simulink subsystem "brakeRegen"  (R2022b)
settings: Solver=VariableStepAuto  StartTime=0.0  StopTime=10.0  RelTol=1e-3
libraries: brakeRegen_lib x1, Raptor_lib x1
settings Model: Creator=serga  LastModifiedBy=serga

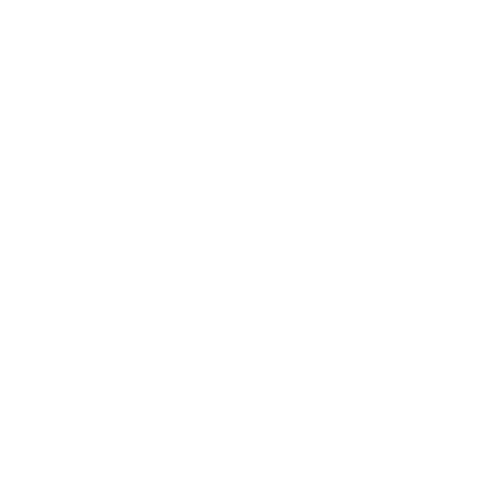
[thumbnail: Simulink's stored preview of the top-level diagram]
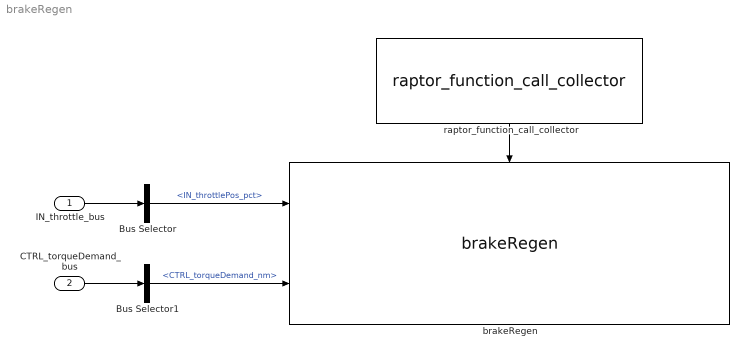
== system brakeRegen ==
  IN_throttle_bus : Inport
  CTRL_torqueDemand_bus : Inport  Port=2
  Bus Selector : BusSelector  OutputSignals=IN_throttlePos_pct
  Bus Selector1 : BusSelector  OutputSignals=CTRL_torqueDemand_nm
  brakeRegen : brakeRegen_lib/brakeRegen  SystemSampleTime=-1  VariantActivationTime=update diagram  Latency=0  AutoFrameSizeCalculation=off
  raptor_function_call_collector : Raptor_lib/Triggers/raptor_function_call_collector  count=5
      settings: SourceProductName=Raptor
  wires:
  raptor_function_call_collector/1 -> brakeRegen/Trigger
  IN_throttle_bus/1 -> Bus Selector/1
  CTRL_torqueDemand_bus/1 -> Bus Selector1/1
  Bus Selector/1 -> brakeRegen/1  "<IN_throttlePos_pct>"
  Bus Selector1/1 -> brakeRegen/2  "<CTRL_torqueDemand_nm>"
